simulink model "controller_sim"  (R2023a)
settings: Solver=VariableStepAuto  StartTime=0.0  StopTime=20  MaxStep=0.01  RelTol=1e-3
values from neighbouring files (symbols this model uses):
  A = [0,    0,    1,    0 ... (first row only)    [controller.m]
  B = [0    0 ... (first row only)    [controller.m]
  C = eye(4)    [controller.m]
  D = zeros(4, 2)    [controller.m]
  K = lqr(A, B(:,1), Q, R)    [controller.m]
settings Model: Creator=ahmed  LastModifiedBy=mahmoudyassermahmoud
settings DebuggingCC: UnconnectedInputMsg=warning  UnconnectedOutputMsg=warning  UnconnectedLineMsg=warning
settings ModelReferenceCC: EnableRefExpFcnMdlSchedulingChecks=on
settings RTWCC: DLArmComputeVersion=19.05

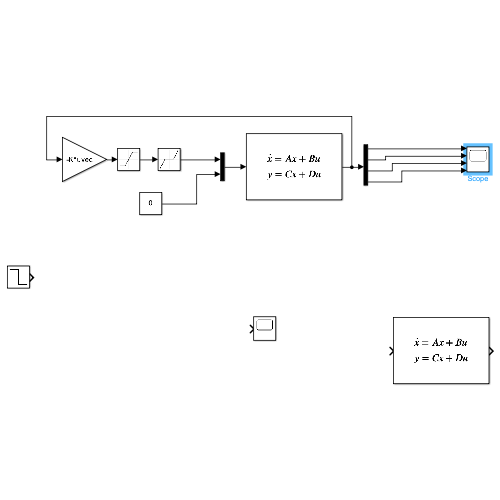
[thumbnail: Simulink's stored preview of the top-level diagram]
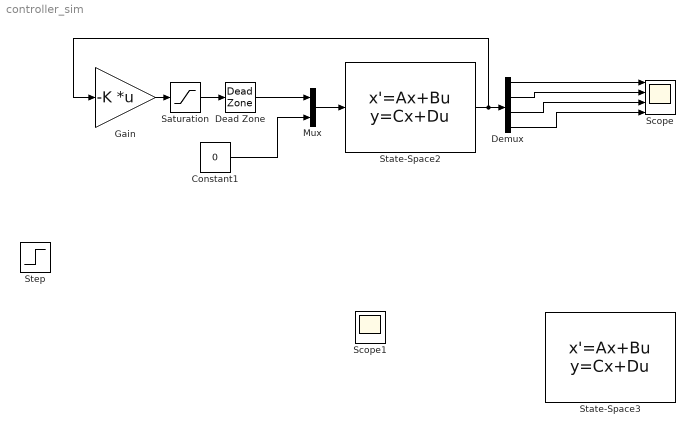
== system controller_sim ==
  Constant1 : Constant  Value=0
  Dead Zone : DeadZone  LowerValue=-2  UpperValue=2
  Demux : Demux
  Gain : Gain  Gain=-K  Multiplication=Matrix(K*u) (u vector)
  Mux : Mux  Inputs=2
  Saturation : Saturate  UpperLimit=12  LowerLimit=-12
  Scope : Scope  NumInputPorts=4
  Scope1 : Scope
  State-Space2 : StateSpace  A=|  B=|  C=C  D=D  InitialCondition=[0;0.2;0;0]  ParameterTunability=Unconstrained
      A=|
      | [0,    0,    1,    0;
      |      0,    0,    0,    1;
      |      0,   (g * m_2^2 * (l2 / 2)^2 * l1 / (((26^2*I+J) + m_2*l1^2) * ( J2_p + m_2*(l2 / 2)^2) - m_2^2 * l1^2 * (l2 / 2)^2)),  (( -b_theta1 * ( J2_p + m_2*(l2 / 2)^2) / (((26^2*I+J) + m_2*l1^2) * ( J2_p + m_2*(l2 / 2)^2) - m_2^2 * l1^2 * (l2 / 2)^2)) - ((( J2_p + m_2*(l2 / 2)^2) / (((26^2*I+J) + m_2*l1^2) * ( J2_p + m_2*(l2 / 2)^2) - m_2^2 * l1^2 * (l2 / 2)^2)) * 26*Kt/r)*(26^2*Kt^2/r)),  (s*-b_theta2 * m_2 * (l2 / 2) * l1 / (((26^2*I+J) + m_2*l1^2) * ( J2_p + m_2*(l2 / 2)^2) - m_2^2 * l1^2 * (l2 / 2)^2));
      |      0,   (s*g * m_2 * (l2 / 2) * ((26^2*I+J) + m_2*l1^2) / (((26^2*I+J) + m_2*l1^2) * ( J2_p + m_2*(l2 / 2)^2) - m_2^2 * l1^2 * (l2 / 2)^2)),  ((s*-b_theta1 * m_2 * (l2 / 2) * l1 / (((26^2*I+J) + m_2*l1^2) * ( J2_p+ m_2*(l2 / 2)^2) - m_2^2 * l1^2 * (l2 / 2)^2)) - ((s*m_2 * (l2 / 2) * l1 / (((26^2*I+J) + m_2*l1^2) * ( J2_p + m_2*(l2 / 2)^2) - m_2^2 * l1^2 * (l2 / 2)^2)) * 26*Kt/r)*(26^2*Kt^2/r)),  (-b_theta2 * ((26^2*I+J) + m_2*l1^2) / (((26^2*I+J) + m_2*l1^2) * ( J2_p + m_2*(l2 / 2)^2) - m_2^2 * l1^2 * (l2 / 2)^2))]
      B=|
      | [0,    0;
      |      0,    0;
      |      ((( J2_p + m_2*(l2 / 2)^2) / (((26^2*I+J) + m_2*l1^2) * ( J2_p + m_2*(l2 / 2)^2) - m_2^2 * l1^2 * (l2 / 2)^2)) * 26*Kt/r),  (s*m_2 * (l2 / 2) * l1 / (((26^2*I+J) + m_2*l1^2) * ( J2_p + m_2*(l2 / 2)^2) - m_2^2 * l1^2 * (l2 / 2)^2));
      |      ((s*m_2 * (l2 / 2) * l1 / (((26^2*I+J) + m_2*l1^2) * ( J2_p + m_2*(l2 / 2)^2) - m_2^2 * l1^2 * (l2 / 2)^2)) * 26*Kt/r),  (((26^2*I+J) + m_2*l1^2) / (((26^2*I+J) + m_2*l1^2) * ( J2_p + m_2*(l2 / 2)^2) - m_2^2 * l1^2 * (l2 / 2)^2))]
  State-Space3 : StateSpace  A=A  B=B  C=C  D=D  InitialCondition=[0;0.2;0;0]  ParameterTunability=Unconstrained
  Step : Step  Time=0.05  Before=150  After=0  SampleTime=0
  wires:
  Demux/1 -> Scope/1
  Demux/2 -> Scope/2
  Demux/4 -> Scope/4
  Demux/3 -> Scope/3
  Constant1/1 -> Mux/2
  Saturation/1 -> Dead Zone/1
  Gain/1 -> Saturation/1
  Mux/1 -> State-Space2/1
  State-Space2/1 -> Gain/1, Demux/1
  Dead Zone/1 -> Mux/1
